simulink model "c28069_offset_T"  (R2018b)
settings: Solver=ode4  StartTime=0.0  StopTime=inf  FixedStep=Tsim  RelTol=1e-3
InitFcn:
  | %Ts=100e-6
  | Tsim = 0.0001
undefined symbols (not defined in the file): serial
libraries: instrumentlib x2, powerlib_meascontrol x1
settings Model: Creator=matti  LastModifiedBy=matti
settings HardwareCC: ProdBitPerPointer=32  ProdBitPerSizeT=32  ProdBitPerPtrDiffT=32  ProdWordSize=32  ProdHWDeviceType=Intel->x86-32 (Windows32)
settings SFSimCC: SimUseLocalCustomCode=off
settings RTWCC: RTWUseLocalCustomCode=off
settings CodeAppCC: StateflowObjectComments=on
settings SimscapeCC: SimscapeNormalizeSystem=off

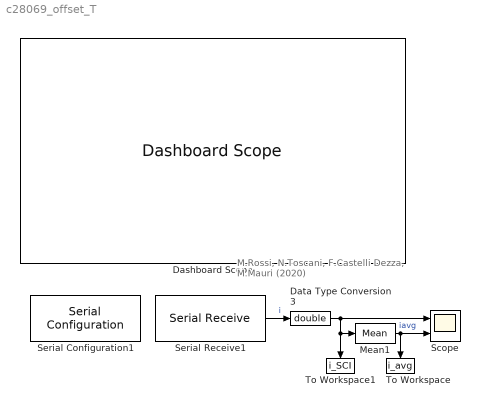
== system c28069_offset_T ==
  note: M.Rossi, N.Toscani, F.Castelli Dezza, M.Mauri (2020)
  Dashboard Scope : DashboardScope  WebBlockId=52  TimeSpan=100  Ymin=-0.10000000000000001  Ymax=1.1000000000000001
  Data Type Conversion3 : DataTypeConversion  OutDataTypeStr=double
  Mean1 : powerlib_meascontrol/Measurements/Mean  Freq=50  Vinit=0  Ts=0
      settings: SourceProductName=Simscape Electrical
  Scope : Scope  NumInputPorts=2
  Serial Configuration1 : instrumentlib/Serial Configuration  Priority=-200000  ComPortMenu=<Please select a port...>  ComPort=COM10  ObjConstructor=serial('COM10');  BaudRate=115200  DataBits=8  Parity=none  StopBits=1  FlowControl=none  Timeout=10  ByteOrder=LittleEndian
  Serial Receive1 : instrumentlib/Serial Receive  ComPortMenu=<Please select a port...>  ComPort=COM10  ObjConstructor=serial('COM10');  Terminator=<none>  DataSize="[1  2]"  DataType=single  EnableBlockingMode=on  ActionDataUnavailable=Output last received value  CustomValue=0  SampleTime=0.01
  To Workspace : ToWorkspace  VariableName=i_avg  SampleTime=0.0001
  To Workspace1 : ToWorkspace  VariableName=i_SCI  SampleTime=0.0001
      settings: Save2DSignal=2-D array (concatenate along first dimension)
  wires:
  Serial Receive1/1 -> Data Type Conversion3/1  "i"
  Mean1/1 -> Scope/2, To Workspace/1  "iavg"
  Data Type Conversion3/1 -> Scope/1, Mean1/1, To Workspace1/1
